simulink model "PRO_TestHarness"  (Simulink 8.6)
settings: Solver=ode45  StartTime=0.0  StopTime=10.0  RelTol=1e-3
PreLoadFcn:
  | addpath('./Workspace/')
  | load('./Workspace/EnvVar.mat')
  | if exist('tl_preloadfcn','file'), tl_preloadfcn(gcs,402); end
PostLoadFcn:
  | if exist('tl_postloadfcn','file'), tl_postloadfcn(gcs,402); end
InitFcn:
  | if exist('tlds_init','file'), tlds_init(gcs); end
StartFcn:
  | if exist('tlds_start','file'), tlds_start(gcs); end
StopFcn:
  | if exist('tlds_stop','file'), tlds_stop(gcs); end
undefined symbols (not defined in the file or in its folder): ddv, sigbuilder_block, Ts
libraries: tllib x19, simulink x2
(part 1 of 5)
PreSaveFcn:
  | if exist('tl_presavefcn','file'), tl_presavefcn(gcs); end
CloseFcn:
  | if exist('tl_closefcn','file'), tl_closefcn(gcs); end
settings Model: TL_MAIN_DATA={'codeopt',{'cleancode',1},'logopt',{'globalloggingmode',4},'date',736811.3266045833,'codegenerationmode',2}  TLRevision=402  DS_PROJECTFILE=PRO_TestHarness.dd  Creator=sabine.flechelle  LastModifiedBy=audrey.vache
settings DataIOCC: SignalLoggingSaveFormat=Dataset
settings OptimizationCC: BlockReduction=off  OptimizeBlockIOStorage=off  BufferReuse=off  GlobalBufferReuse=off  ExpressionFolding=off  ExpressionDepthLimit=128  LocalBlockOutputs=off
settings DebuggingCC: FcnCallInpInsideContextMsg=UseLocalSettings  BusObjectLabelMismatch=error  StateNameClashWarn=none  StrictBusMsg=ErrorOnBusTreatedAsVector  NonBusSignalsTreatedAsBus=error

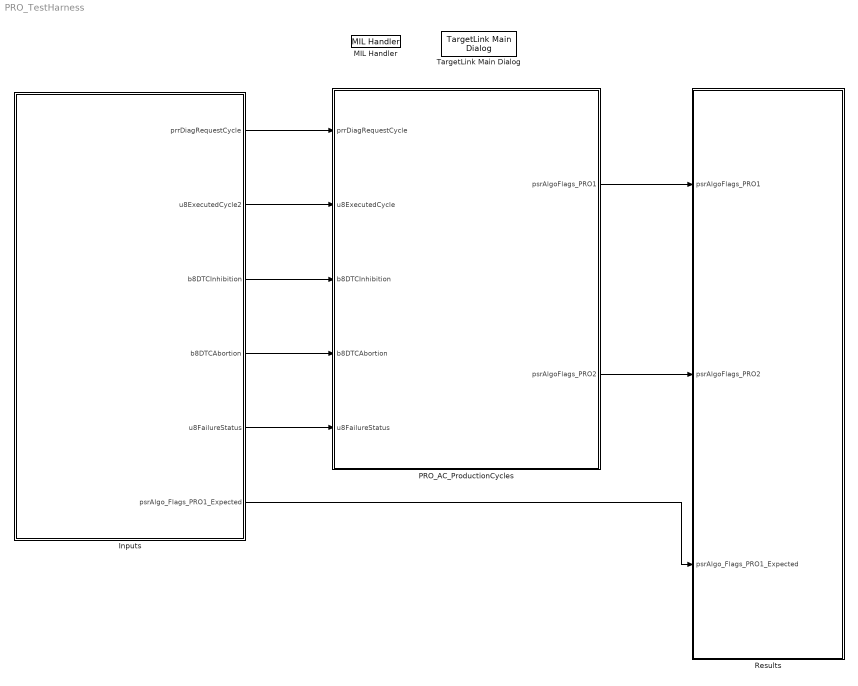
== system PRO_TestHarness ==
  Inputs : Subsystem
  MIL Handler : tllib/MIL Handler  data={'date',730486}
  PRO_AC_ProductionCycles : Subsystem  Tag=TargetLink Simulation Frame  mask(TL_SimFrame){}
      settings: CopyFcn=if exist('tl_copyfcn','file'), tl_copyfcn(gcbh); end  NameChangeFcn=if exist('tl_framenamechangefcn','file'), tl_framenamechangefcn(gcbh); end
      settings: OpenFcn=|
      | if exist('open_tlsubsystem','file')
      |    open_tlsubsystem(gcbh);
      | else
      |    tlsubsystem = ...
      |       find_system(gcb, ...
      |       'LookUnderMasks','on', ...
      |       'FollowLinks','on', ...
      |       'Tag','MIL Subsystem');
      |    open_system(tlsubsystem);
      | end
      mask Display: disp('TargetLink\nSoftware-\nin-the-loop\nmode')
  Results : Subsystem
  TargetLink Main Dialog : tllib/TargetLink Main Dialog  data=[]
  wires:
  Inputs/3(b8DTCInhibition) -> PRO_AC_ProductionCycles/3(b8DTCInhibition)
  Inputs/4(b8DTCAbortion) -> PRO_AC_ProductionCycles/4(b8DTCAbortion)
  Inputs/2(u8ExecutedCycle2) -> PRO_AC_ProductionCycles/2(u8ExecutedCycle)
  PRO_AC_ProductionCycles/1(psrAlgoFlags_PRO1) -> Results/1(psrAlgoFlags_PRO1)
  Inputs/6(psrAlgo_Flags_PRO1_Expected) -> Results/3(psrAlgo_Flags_PRO1_Expected)
  Inputs/1(prrDiagRequestCycle) -> PRO_AC_ProductionCycles/1(prrDiagRequestCycle)
  PRO_AC_ProductionCycles/2(psrAlgoFlags_PRO2) -> Results/2(psrAlgoFlags_PRO2)
  Inputs/5(u8FailureStatus) -> PRO_AC_ProductionCycles/5(u8FailureStatus)

== system PRO_TestHarness/Inputs ==
  Bus Creator1 : BusCreator  Inputs=2
  Bus Creator3 : BusCreator  Inputs=1
  BusCreator : BusCreator  Inputs=5
  Constant1 : Constant  Value=ddv('BFD/KU8_ZERO')  OutDataTypeStr=uint8  mask(TL_Constant){data={'output',{'variable','BFD/KU8_ZERO'},'date',736231.40062822914}}
      settings: DeleteFcn=if exist('delete_tlblock','file')==2,delete_tlblock(gcbh);end  NameChangeFcn=if exist('rename_tlblock','file')==2,rename_tlblock(gcbh);end  OpenFcn=if exist('tl_open_blockdlg','file')==2,tl_open_blockdlg(gcbh);else,open_system(gcbh,'parameter');end
      mask Help: eval(['if exist(''tl_online_help'',''file'') == 2, tl_online_help(''Topic'',''TL_Constant''),else, web([''jar:file:///'',matlabroot,''/help/toolbox/simulink/help.jar!/slref/' lower(get_param(gcbh,'Blocktype')) '.html''], ''-helpbrowser''),end'])
      mask Display: plot([-0.05, 1.05, NaN, -0.05, 1.05],[.01, .01, NaN, .99, .99])
  Manage_Sampling : Subsystem  TreatAsAtomicUnit=on
  Signal Builder : Subsystem  Tag=STV Subsys  LoadFcn=sigbuilder_block('load');  StartFcn=sigbuilder_block('start');  StopFcn=sigbuilder_block('stop');  ClipboardFcn=sigbuilder_block('clipboard');  mask(Sigbuilder block){}
      mask init:
      | if ~strcmp(get_param(bdroot(gcb),'SimulationStatus'),'stopped') tuvar = sigbuilder_block('maskInit'); end
      settings: CopyFcn=sigbuilder_block('copy');  DeleteFcn=sigbuilder_block('delete');  ModelCloseFcn=sigbuilder_block('modelClose');  PreSaveFcn=sigbuilder_block('preSave');  PauseFcn=sigbuilder_block('pause')  ContinueFcn=sigbuilder_block('continue')  NameChangeFcn=sigbuilder_block('namechange');  OpenFcn=sigbuilder_block('open',[132.75 123 813.75 406.5 ]);  CloseFcn=sigbuilder_block('close');
      mask Display: plot(0,0,100,100,[10,10,40,40,10],[80,20,20,80,80],[40,10],[50,50], [40,27,10],[65,72,56],[40,25,25,10],[28,28,43,43]);
  Terminator : Terminator
  prrDiagRequestCycle : Outport
  u8ExecutedCycle2 : Outport  Port=2  OutDataTypeStr=uint8  PortDimensions=1
  b8DTCInhibition : Outport  Port=3  PortDimensions=1
  b8DTCAbortion : Outport  Port=4  PortDimensions=1
  u8FailureStatus : Outport  Port=5
  psrAlgo_Flags_PRO1_Expected : Outport  Port=6
  wires:
  Manage_Sampling/4(b8DTCInhibition) -> b8DTCInhibition/1
  Manage_Sampling/3(u8ExecutedCycle2) -> u8ExecutedCycle2/1
  Manage_Sampling/5(b8DTCAbortion) -> b8DTCAbortion/1
  Bus Creator3/1 -> prrDiagRequestCycle/1
  Manage_Sampling/1(u8RequestedCycle1) -> Bus Creator3/1  "u8RequestedCycle"
  Manage_Sampling/2(u8RequestedCycleComplement1) -> Terminator/1  "u8RequestedCycleComplement"
  BusCreator/1 -> psrAlgo_Flags_PRO1_Expected/1
  Manage_Sampling/7(b8TriggeringOrder_Expected2) -> BusCreator/1
  Manage_Sampling/8(b8AbortionOrder_Expected2) -> BusCreator/2
  Manage_Sampling/9(b8PreActivationFlag_Expected1) -> BusCreator/3
  Manage_Sampling/10(b8PreConditionsFlag_Expected) -> BusCreator/4
  Manage_Sampling/11(u8TriggeringSource_Expected5) -> BusCreator/5
  Signal Builder/11(u8TriggeringSource_PRO1_Expected) -> Manage_Sampling/11(u8TriggeringSource_Expected4)
  Signal Builder/10(b8PreConditionsFlag_PRO1_Expected) -> Manage_Sampling/10(b8PreConditionsFlag_Expected2)
  Signal Builder/5(bAbortionMode) -> Manage_Sampling/5(b8DTCAbortion1)
  Signal Builder/3(u8ExecutedCycle) -> Manage_Sampling/3(u8ExecutedCycle)
  Signal Builder/4(btInhibitionMode) -> Manage_Sampling/4(b8DTCInhibition1)
  Signal Builder/8(b8AbortionFlag_PRO1_Expected) -> Manage_Sampling/8(b8AbortionOrder_Expected)
  Signal Builder/7(b8TriggerFlag_PRO1_Expected) -> Manage_Sampling/7(b8TriggeringOrder_Expected)
  Signal Builder/2(u8RequestedCycleComplement) -> Manage_Sampling/2(u8RequestedCycleComplement)
  Signal Builder/9(b8PreActivationFlag_PRO1_Expected) -> Manage_Sampling/9(b8PreActivationFlag_Expected)
  Signal Builder/1(u8RequestedCycle) -> Manage_Sampling/1(u8RequestedCycle)
  Bus Creator1/1 -> u8FailureStatus/1
  Constant1/1 -> Bus Creator1/1  "u8Status_UVDuringTensioning"
  Manage_Sampling/6(b8OverVoltageStatus1) -> Bus Creator1/2  "u8Status_OverVoltage"
  Signal Builder/6(b8OverVoltageStatus) -> Manage_Sampling/6(b8OverVoltageStatus)

== system PRO_TestHarness/PRO_AC_ProductionCycles ==
  prrDiagRequestCycle : Inport
  u8ExecutedCycle : Inport  Port=2
  b8DTCInhibition : Inport  Port=3  OutDataTypeStr=uint8
  b8DTCAbortion : Inport  Port=4  OutDataTypeStr=uint8
  u8FailureStatus : Inport  Port=5
  S-function frame : Subsystem
  Subsystem : Subsystem  Tag=struct('sfcnName','PRO_AC_ProductionCycles_sf','subFunction','','srcSubsystem','')  Commented=on  mask(TL_Enable){}
      settings: OpenFcn=warndlg(get_param(gcb,'MaskHelp'),'Serious Warning');
      mask Help: This subsystem keeps the TargetLink subsystem (subsystem with TargetLink blocks for production code generation), and is needed for the TargetLink simulation frame to work properly. DO NOT DELETE OR MODIFY IT!
  Timer : simulink/Ports & Subsystems/Function-Call Generator  sample_time=0.01  numberOfIterations=1
  psrAlgoFlags_PRO1 : Outport
  psrAlgoFlags_PRO2 : Outport  Port=2
  wires:
  Timer/1 -> S-function frame/Trigger
  prrDiagRequestCycle/1 -> S-function frame/1(In1)
  u8ExecutedCycle/1 -> S-function frame/2(In2)
  b8DTCInhibition/1 -> S-function frame/3(In3)
  b8DTCAbortion/1 -> S-function frame/4(In4)
  u8FailureStatus/1 -> S-function frame/5(In5)
  S-function frame/1(Out1) -> psrAlgoFlags_PRO1/1
  S-function frame/2(Out2) -> psrAlgoFlags_PRO2/1

== system PRO_TestHarness/Results ==
  psrAlgoFlags_PRO1 : Inport
  psrAlgoFlags_PRO2 : Inport  Port=2
  psrAlgo_Flags_PRO1_Expected : Inport  Port=3
  BusSelector1 : BusSelector  OutputSignals=b8TriggerFlag_PR01,b8InterruptFlag_PRO1,b8PreActivationFlag_PRO1,b8PreConditionsFlag_PRO1,u8TriggeringSource_PRO1
  BusSelector3 : BusSelector  OutputSignals=b8TriggerFlag_PRO2,b8InterruptFlag_PRO2,b8ActivationFlag_PRO2,b8PreConditionsFlag_PRO2,u8TriggeringSource_PRO2
  Data Type Conversion{,1,4,8..12,19..20} (10 alike) : DataTypeConversion  OutDataTypeStr=double  RndMeth=Nearest
  Mux : Mux  Inputs=10
  Scope : Scope  NumInputPorts=5
  To Workspace : ToWorkspace  VariableName=Simout  SaveFormat=Structure  SampleTime=-1
  wires:
  psrAlgoFlags_PRO1/1 -> BusSelector1/1
  BusSelector1/1 -> Scope/1, Data Type Conversion/1  "<b8TriggerFlag_PR01>"
  BusSelector1/2 -> Scope/2, Data Type Conversion1/1  "<b8InterruptFlag_PRO1>"
  Data Type Conversion/1 -> Mux/1
  Data Type Conversion1/1 -> Mux/2
  Data Type Conversion4/1 -> Mux/3
  Mux/1 -> To Workspace/1
  Data Type Conversion19/1 -> Mux/4
  Data Type Conversion20/1 -> Mux/5
  BusSelector1/3 -> Scope/3, Data Type Conversion4/1  "<b8PreActivationFlag_PRO1>"
  BusSelector1/4 -> Scope/4, Data Type Conversion19/1  "<b8PreConditionsFlag_PRO1>"
  BusSelector1/5 -> Scope/5, Data Type Conversion20/1  "<u8TriggeringSource_PRO1>"
  BusSelector3/1 -> Data Type Conversion8/1  "<b8TriggerFlag_PRO2>"
  BusSelector3/2 -> Data Type Conversion9/1  "<b8InterruptFlag_PRO2>"
  BusSelector3/3 -> Data Type Conversion12/1  "<b8ActivationFlag_PRO2>"
  BusSelector3/4 -> Data Type Conversion10/1  "<b8PreConditionsFlag_PRO2>"
  BusSelector3/5 -> Data Type Conversion11/1  "<u8TriggeringSource_PRO2>"
  psrAlgoFlags_PRO2/1 -> BusSelector3/1
  Data Type Conversion9/1 -> Mux/7
  Data Type Conversion8/1 -> Mux/6
  Data Type Conversion10/1 -> Mux/9
  Data Type Conversion11/1 -> Mux/10
  Data Type Conversion12/1 -> Mux/8

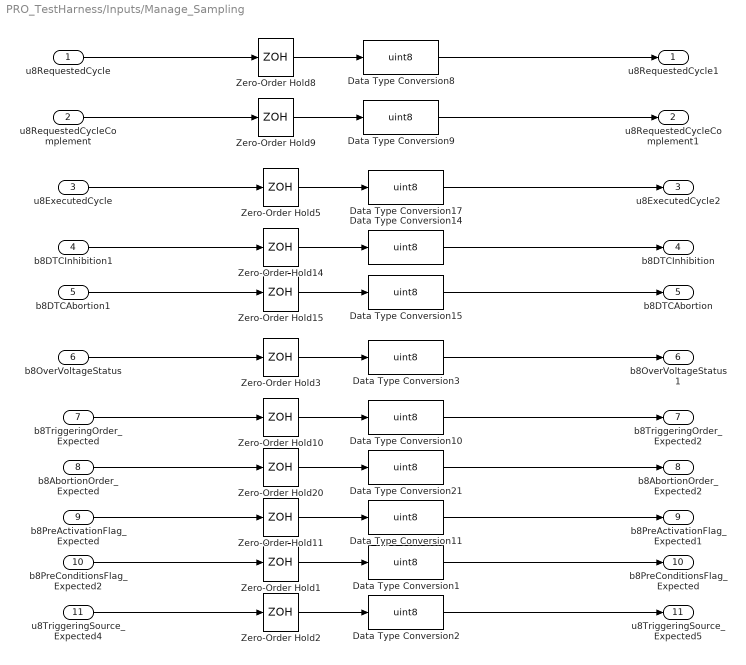
== system PRO_TestHarness/Inputs/Manage_Sampling ==
  u8RequestedCycle : Inport
      settings: NameChangeFcn=if exist('tl_check_ports','file'), tl_check_ports(gcbh); end
      settings: CopyFcn=|
      | if exist('tl_reset_reviewflag','file')==2
      |     tl_reset_reviewflag(gcbh);
      | end
      | if exist('tl_check_ports','file')
      |     tl_check_ports(gcbh);
      | end
  u8RequestedCycleComplement : Inport  Port=2
      settings: NameChangeFcn=if exist('tl_check_ports','file'), tl_check_ports(gcbh); end
      settings: CopyFcn=|
      | if exist('tl_reset_reviewflag','file')==2
      |     tl_reset_reviewflag(gcbh);
      | end
      | if exist('tl_check_ports','file')
      |     tl_check_ports(gcbh);
      | end
  u8ExecutedCycle : Inport  Port=3
      settings: NameChangeFcn=if exist('tl_check_ports','file'), tl_check_ports(gcbh); end
      settings: CopyFcn=|
      | if exist('tl_reset_reviewflag','file')==2
      |     tl_reset_reviewflag(gcbh);
      | end
      | if exist('tl_check_ports','file')
      |     tl_check_ports(gcbh);
      | end
  b8DTCInhibition1 : Inport  Port=4
      settings: NameChangeFcn=if exist('tl_check_ports','file'), tl_check_ports(gcbh); end
      settings: CopyFcn=|
      | if exist('tl_reset_reviewflag','file')==2
      |     tl_reset_reviewflag(gcbh);
      | end
      | if exist('tl_check_ports','file')
      |     tl_check_ports(gcbh);
      | end
  b8DTCAbortion1 : Inport  Port=5
      settings: NameChangeFcn=if exist('tl_check_ports','file'), tl_check_ports(gcbh); end
      settings: CopyFcn=|
      | if exist('tl_reset_reviewflag','file')==2
      |     tl_reset_reviewflag(gcbh);
      | end
      | if exist('tl_check_ports','file')
      |     tl_check_ports(gcbh);
      | end
  b8OverVoltageStatus : Inport  Port=6
      settings: NameChangeFcn=if exist('tl_check_ports','file'), tl_check_ports(gcbh); end
      settings: CopyFcn=|
      | if exist('tl_reset_reviewflag','file')==2
      |     tl_reset_reviewflag(gcbh);
      | end
      | if exist('tl_check_ports','file')
      |     tl_check_ports(gcbh);
      | end
  b8TriggeringOrder_Expected : Inport  Port=7
  b8AbortionOrder_Expected : Inport  Port=8
  b8PreActivationFlag_Expected : Inport  Port=9
  b8PreConditionsFlag_Expected2 : Inport  Port=10
  u8TriggeringSource_Expected4 : Inport  Port=11
  Data Type Conversion{1..3,8..11,14..15,17,21} (11 alike) : DataTypeConversion  OutDataTypeStr=uint8
  Zero-Order Hold{1..3,5,8..11,14..15,20} (11 alike) : ZeroOrderHold  SampleTime=Ts
  u8RequestedCycle1 : Outport  PortDimensions=1
  u8RequestedCycleComplement1 : Outport  Port=2  PortDimensions=1
  u8ExecutedCycle2 : Outport  Port=3  PortDimensions=1
  b8DTCInhibition : Outport  Port=4  PortDimensions=1
  b8DTCAbortion : Outport  Port=5  PortDimensions=1
  b8OverVoltageStatus1 : Outport  Port=6  PortDimensions=1
  b8TriggeringOrder_Expected2 : Outport  Port=7
  b8AbortionOrder_Expected2 : Outport  Port=8
  b8PreActivationFlag_Expected1 : Outport  Port=9
  b8PreConditionsFlag_Expected : Outport  Port=10
  u8TriggeringSource_Expected5 : Outport  Port=11
  wires:
  Data Type Conversion15/1 -> b8DTCAbortion/1
  Data Type Conversion14/1 -> b8DTCInhibition/1
  b8DTCAbortion1/1 -> Zero-Order Hold15/1
  Zero-Order Hold15/1 -> Data Type Conversion15/1
  b8DTCInhibition1/1 -> Zero-Order Hold14/1
  Zero-Order Hold14/1 -> Data Type Conversion14/1
  Data Type Conversion17/1 -> u8ExecutedCycle2/1
  u8ExecutedCycle/1 -> Zero-Order Hold5/1
  Zero-Order Hold5/1 -> Data Type Conversion17/1
  Zero-Order Hold10/1 -> Data Type Conversion10/1
  Zero-Order Hold11/1 -> Data Type Conversion11/1
  b8TriggeringOrder_Expected/1 -> Zero-Order Hold10/1
  Data Type Conversion10/1 -> b8TriggeringOrder_Expected2/1
  Zero-Order Hold20/1 -> Data Type Conversion21/1
  Data Type Conversion11/1 -> b8PreActivationFlag_Expected1/1
  Data Type Conversion21/1 -> b8AbortionOrder_Expected2/1
  b8AbortionOrder_Expected/1 -> Zero-Order Hold20/1
  b8PreActivationFlag_Expected/1 -> Zero-Order Hold11/1
  Data Type Conversion8/1 -> u8RequestedCycle1/1
  u8RequestedCycle/1 -> Zero-Order Hold8/1
  Zero-Order Hold8/1 -> Data Type Conversion8/1
  Data Type Conversion9/1 -> u8RequestedCycleComplement1/1
  u8RequestedCycleComplement/1 -> Zero-Order Hold9/1
  Zero-Order Hold9/1 -> Data Type Conversion9/1
  Zero-Order Hold1/1 -> Data Type Conversion1/1
  Data Type Conversion1/1 -> b8PreConditionsFlag_Expected/1
  b8PreConditionsFlag_Expected2/1 -> Zero-Order Hold1/1
  Zero-Order Hold2/1 -> Data Type Conversion2/1
  Data Type Conversion2/1 -> u8TriggeringSource_Expected5/1
  u8TriggeringSource_Expected4/1 -> Zero-Order Hold2/1
  Data Type Conversion3/1 -> b8OverVoltageStatus1/1
  b8OverVoltageStatus/1 -> Zero-Order Hold3/1
  Zero-Order Hold3/1 -> Data Type Conversion3/1

== system PRO_TestHarness/Inputs/Signal Builder ==
  Demux : Demux  Tag=STV Demux  Outputs=11
  FromWs : FromWorkspace  Tag=STV FromWs  VariableName=tuvar  SampleTime=0.01  Interpolate=off  OutputAfterFinalValue=Holding final value  SigBuilderData=DataTag0  VnvData=DataTag1
      SigBuilderData=|
      | dataSet(1).timeRange = [0 10]
      | dataSet(1).name = 'Template_Tests'
      | dataSet(2).timeRange = [0 10]
      | dataSet(2).name = 'MBD_PRO_01_Nominal'
      | dataSet(3).timeRange = [0 10]
      | dataSet(3).name = 'MBD_PRO_01_Nominal1'
      | dataSet(4).timeRange = [0 10]
      | dataSet(4).name = 'MBD_PRO_01_Nominal2'
      | sbobj.Name = 'Signal Builder'
      | sbobj.Groups(1).Name = 'Template_Tests'
      | sbobj.Groups(1).Signals(1).Name = 'u8RequestedCycle'
      | sbobj.Groups(1).Signals(1).XData = [0 10]
      | sbobj.Groups(1).Signals(1).YData = [0 0]
      | sbobj.Groups(1).Signals(2).Name = 'u8RequestedCycleComplement'
      | sbobj.Groups(1).Signals(2).XData = [0 10]
      | sbobj.Groups(1).Signals(2).YData = [0 0]
      | sbobj.Groups(1).Signals(3).Name = 'u8ExecutedCycle'
      | sbobj.Groups(1).Signals(3).XData = [0 10]
      | sbobj.Groups(1).Signals(3).YData = [0 0]
      | sbobj.Groups(1).Signals(4).Name = 'btInhibitionMode'
      | sbobj.Groups(1).Signals(4).XData = [0 10]
      | sbobj.Groups(1).Signals(4).YData = [0 0]
      | sbobj.Groups(1).Signals(5).Name = 'bAbortionMode'
      | sbobj.Groups(1).Signals(5).XData = [0 10]
      | sbobj.Groups(1).Signals(5).YData = [0 0]
      | sbobj.Groups(1).Signals(6).Name = 'b8OverVoltageStatus'
      | sbobj.Groups(1).Signals(6).XData = [0 10]
      | sbobj.Groups(1).Signals(6).YData = [0 0]
      | sbobj.Groups(1).Signals(7).Name = 'b8TriggerFlag_PRO1_Expected'
      | sbobj.Groups(1).Signals(7).XData = [0 10]
      | sbobj.Groups(1).Signals(7).YData = [0 0]
      | sbobj.Groups(1).Signals(8).Name = 'b8AbortionFlag_PRO1_Expected'
      | sbobj.Groups(1).Signals(8).XData = [0 10]
      | sbobj.Groups(1).Signals(8).YData = [0 0]
      | sbobj.Groups(1).Signals(9).Name = 'b8PreActivationFlag_PRO1_Expected'
      | sbobj.Groups(1).Signals(9).XData = [0 10]
      | sbobj.Groups(1).Signals(9).YData = [0 0]
      | sbobj.Groups(1).Signals(10).Name = 'b8PreConditionsFlag_PRO1_Expected'
      | sbobj.Groups(1).Signals(10).XData = [0 10]
      | sbobj.Groups(1).Signals(10).YData = [0 0]
      | sbobj.Groups(1).Signals(11).Name = 'u8TriggeringSource_PRO1_Expected'
      | sbobj.Groups(1).Signals(11).XData = [0 10]
      | sbobj.Groups(1).Signals(11).YData = [0 0]
      | sbobj.Groups(2).Name = 'MBD_PRO_01_Nominal'
      | sbobj.Groups(2).Signals(1).Name = 'u8RequestedCycle'
      | sbobj.Groups(2).Signals(1).XData = [0 0.009 0.009 0.019 0.019 0.029 0.029 0.039 0.039 0.049 0.049 0.059 ... (2000 elements, 1x2000)]
      | sbobj.Groups(2).Signals(1).YData = [255 255 255 255 255 255 255 255 255 255 255 255 ... (2000 elements, 1x2000)]
      | sbobj.Groups(2).Signals(2).Name = 'u8RequestedCycleComplement'
      | sbobj.Groups(2).Signals(2).XData = [0 0.009 0.009 0.019 0.019 0.029 0.029 0.039 0.039 0.049 0.049 0.059 ... (2000 elements, 1x2000)]
      | sbobj.Groups(2).Signals(2).YData = [0 0 0 0 0 0 0 0 0 0 0 0 ... (2000 elements, 1x2000)]
      | sbobj.Groups(2).Signals(3).Name = 'u8ExecutedCycle'
      | sbobj.Groups(2).Signals(3).XData = [0 0.009 0.009 0.019 0.019 0.029 0.029 0.039 0.039 0.049 0.049 0.059 ... (2000 elements, 1x2000)]
      | sbobj.Groups(2).Signals(3).YData = [255 255 255 255 255 255 255 255 255 255 255 255 ... (2000 elements, 1x2000)]
      | sbobj.Groups(2).Signals(4).Name = 'btInhibitionMode'
      | sbobj.Groups(2).Signals(4).XData = [0 0.009 0.009 0.019 0.019 0.029 0.029 0.039 0.039 0.049 0.049 0.059 ... (2000 elements, 1x2000)]
      | sbobj.Groups(2).Signals(4).YData = [85 85 85 85 85 85 85 85 85 85 85 85 ... (2000 elements, 1x2000)]
      | sbobj.Groups(2).Signals(5).Name = 'bAbortionMode'
      | sbobj.Groups(2).Signals(5).XData = [0 0.009 0.009 0.019 0.019 0.029 0.029 0.039 0.039 0.049 0.049 0.059 ... (2000 elements, 1x2000)]
      | sbobj.Groups(2).Signals(5).YData = [85 85 85 85 85 85 85 85 85 85 85 85 ... (2000 elements, 1x2000)]
      | sbobj.Groups(2).Signals(6).Name = 'b8OverVoltageStatus'
      | sbobj.Groups(2).Signals(6).XData = [0 0.009 0.009 0.019 0.019 0.029 0.029 0.039 0.039 0.049 0.049 0.059 ... (2000 elements, 1x2000)]
      | sbobj.Groups(2).Signals(6).YData = [0 0 0 0 0 0 0 0 0 0 0 0 ... (2000 elements, 1x2000)]
      | sbobj.Groups(2).Signals(7).Name = 'b8TriggerFlag_PRO1_Expected'
      | sbobj.Groups(2).Signals(7).XData = [0 0.009 0.009 0.019 0.019 0.029 0.029 0.039 0.039 0.049 0.049 0.059 ... (2000 elements, 1x2000)]
      | sbobj.Groups(2).Signals(7).YData = [85 85 85 85 85 85 85 85 85 85 85 85 ... (2000 elements, 1x2000)]
      | sbobj.Groups(2).Signals(8).Name = 'b8AbortionFlag_PRO1_Expected'
      | sbobj.Groups(2).Signals(8).XData = [0 0.009 0.009 0.019 0.019 0.029 0.029 0.039 0.039 0.049 0.049 0.059 ... (2000 elements, 1x2000)]
      | sbobj.Groups(2).Signals(8).YData = [85 85 85 85 85 85 85 85 85 85 85 85 ... (2000 elements, 1x2000)]
      | sbobj.Groups(2).Signals(9).Name = 'b8PreActivationFlag_PRO1_Expected'
      | sbobj.Groups(2).Signals(9).XData = [0 0.009 0.009 0.019 0.019 0.029 0.029 0.039 0.039 0.049 0.049 0.059 ... (2000 elements, 1x2000)]
      | sbobj.Groups(2).Signals(9).YData = [85 85 85 85 85 85 85 85 85 85 85 85 ... (2000 elements, 1x2000)]
      | sbobj.Groups(2).Signals(10).Name = 'b8PreConditionsFlag_PRO1_Expected'
      | sbobj.Groups(2).Signals(10).XData = [0 0.009 0.009 0.019 0.019 0.029 0.029 0.039 0.039 0.049 0.049 0.059 ... (2000 elements, 1x2000)]
      | sbobj.Groups(2).Signals(10).YData = [170 170 170 170 170 170 170 170 170 170 170 170 ... (2000 elements, 1x2000)]
      | sbobj.Groups(2).Signals(11).Name = 'u8TriggeringSource_PRO1_Expected'
      | sbobj.Groups(2).Signals(11).XData = [0 0.009 0.009 0.019 0.019 0.029 0.029 0.039 0.039 0.049 0.049 0.059 ... (2000 elements, 1x2000)]
      | sbobj.Groups(2).Signals(11).YData = [0 0 0 0 0 0 0 0 0 0 0 0 ... (2000 elements, 1x2000)]
      | sbobj.Groups(3).Name = 'MBD_PRO_01_Nominal1'
      | sbobj.Groups(3).Signals(1).Name = 'u8RequestedCycle'
      | sbobj.Groups(3).Signals(1).XData = [0 0.009 0.009 0.019 0.019 0.029 0.029 0.039 0.039 0.049 0.049 0.059 ... (2000 elements, 1x2000)]
      | sbobj.Groups(3).Signals(1).YData = [255 255 255 255 255 255 255 255 255 255 255 255 ... (2000 elements, 1x2000)]
      | sbobj.Groups(3).Signals(2).Name = 'u8RequestedCycleComplement'
      | sbobj.Groups(3).Signals(2).XData = [0 0.009 0.009 0.019 0.019 0.029 0.029 0.039 0.039 0.049 0.049 0.059 ... (2000 elements, 1x2000)]
      | sbobj.Groups(3).Signals(2).YData = [0 0 0 0 0 0 0 0 0 0 0 0 ... (2000 elements, 1x2000)]
      | sbobj.Groups(3).Signals(3).Name = 'u8ExecutedCycle'
      | sbobj.Groups(3).Signals(3).XData = [0 0.009 0.009 0.019 0.019 0.029 0.029 0.039 0.039 0.049 0.049 0.059 ... (2000 elements, 1x2000)]
      | sbobj.Groups(3).Signals(3).YData = [255 255 255 255 255 255 255 255 255 255 255 255 ... (2000 elements, 1x2000)]
      | sbobj.Groups(3).Signals(4).Name = 'btInhibitionMode'
      | sbobj.Groups(3).Signals(4).XData = [0 0.009 0.009 0.019 0.019 0.029 0.029 0.039 0.039 0.049 0.049 0.059 ... (2000 elements, 1x2000)]
      | sbobj.Groups(3).Signals(4).YData = [85 85 85 85 85 85 85 85 85 85 85 85 ... (2000 elements, 1x2000)]
      | sbobj.Groups(3).Signals(5).Name = 'bAbortionMode'
      | sbobj.Groups(3).Signals(5).XData = [0 0.009 0.009 0.019 0.019 0.029 0.029 0.039 0.039 0.049 0.049 0.059 ... (2000 elements, 1x2000)]
      | sbobj.Groups(3).Signals(5).YData = [85 85 85 85 85 85 85 85 85 85 85 85 ... (2000 elements, 1x2000)]
      | sbobj.Groups(3).Signals(6).Name = 'b8OverVoltageStatus'
      | sbobj.Groups(3).Signals(6).XData = [0 0.009 0.009 0.019 0.019 0.029 0.029 0.039 0.039 0.049 0.049 0.059 ... (2000 elements, 1x2000)]
      | sbobj.Groups(3).Signals(6).YData = [0 0 0 0 0 0 0 0 0 0 0 0 ... (2000 elements, 1x2000)]
      | sbobj.Groups(3).Signals(7).Name = 'b8TriggerFlag_PRO1_Expected'
      | sbobj.Groups(3).Signals(7).XData = [0 0.009 0.009 0.019 0.019 0.029 0.029 0.039 0.039 0.049 0.049 0.059 ... (2000 elements, 1x2000)]
      | sbobj.Groups(3).Signals(7).YData = [85 85 85 85 85 85 85 85 85 85 85 85 ... (2000 elements, 1x2000)]
      | sbobj.Groups(3).Signals(8).Name = 'b8AbortionFlag_PRO1_Expected'
      | sbobj.Groups(3).Signals(8).XData = [0 0.009 0.009 0.019 0.019 0.029 0.029 0.039 0.039 0.049 0.049 0.059 ... (2000 elements, 1x2000)]
      | sbobj.Groups(3).Signals(8).YData = [85 85 85 85 85 85 85 85 85 85 85 85 ... (2000 elements, 1x2000)]
      | sbobj.Groups(3).Signals(9).Name = 'b8PreActivationFlag_PRO1_Expected'
      | sbobj.Groups(3).Signals(9).XData = [0 0.009 0.009 0.019 0.019 0.029 0.029 0.039 0.039 0.049 0.049 0.059 ... (2000 elements, 1x2000)]
      | sbobj.Groups(3).Signals(9).YData = [85 85 85 85 85 85 85 85 85 85 85 85 ... (2000 elements, 1x2000)]
      | sbobj.Groups(3).Signals(10).Name = 'b8PreConditionsFlag_PRO1_Expected'
      | sbobj.Groups(3).Signals(10).XData = [0 0.009 0.009 0.019 0.019 0.029 0.029 0.039 0.039 0.049 0.049 0.059 ... (2000 elements, 1x2000)]
      | sbobj.Groups(3).Signals(10).YData = [170 170 170 170 170 170 170 170 170 170 170 170 ... (2000 elements, 1x2000)]
      | sbobj.Groups(3).Signals(11).Name = 'u8TriggeringSource_PRO1_Expected'
      | sbobj.Groups(3).Signals(11).XData = [0 0.009 0.009 0.019 0.019 0.029 0.029 0.039 0.039 0.049 0.049 0.059 ... (2000 elements, 1x2000)]
      | sbobj.Groups(3).Signals(11).YData = [0 0 0 0 0 0 0 0 0 0 0 0 ... (2000 elements, 1x2000)]
      | sbobj.Groups(4).Name = 'MBD_PRO_01_Nominal2'
      | sbobj.Groups(4).Signals(1).Name = 'u8RequestedCycle'
      | sbobj.Groups(4).Signals(1).XData = [0 0.009 0.009 0.019 0.019 0.029 0.029 0.039 0.039 0.049 0.049 0.059 ... (2000 elements, 1x2000)]
      | sbobj.Groups(4).Signals(1).YData = [255 255 255 255 255 255 255 255 255 255 255 255 ... (2000 elements, 1x2000)]
      | sbobj.Groups(4).Signals(2).Name = 'u8RequestedCycleComplement'
      | sbobj.Groups(4).Signals(2).XData = [0 0.009 0.009 0.019 0.019 0.029 0.029 0.039 0.039 0.049 0.049 0.059 ... (2000 elements, 1x2000)]
      | sbobj.Groups(4).Signals(2).YData = [0 0 0 0 0 0 0 0 0 0 0 0 ... (2000 elements, 1x2000)]
      | sbobj.Groups(4).Signals(3).Name = 'u8ExecutedCycle'
      | sbobj.Groups(4).Signals(3).XData = [0 0.009 0.009 0.019 0.019 0.029 0.029 0.039 0.039 0.049 0.049 0.059 ... (2000 elements, 1x2000)]
      | sbobj.Groups(4).Signals(3).YData = [255 255 255 255 255 255 255 255 255 255 255 255 ... (2000 elements, 1x2000)]
      | sbobj.Groups(4).Signals(4).Name = 'btInhibitionMode'
      | sbobj.Groups(4).Signals(4).XData = [0 0.009 0.009 0.019 0.019 0.029 0.029 0.039 0.039 0.049 0.049 0.059 ... (2000 elements, 1x2000)]
      | sbobj.Groups(4).Signals(4).YData = [85 85 85 85 85 85 85 85 85 85 85 85 ... (2000 elements, 1x2000)]
      | sbobj.Groups(4).Signals(5).Name = 'bAbortionMode'
      | sbobj.Groups(4).Signals(5).XData = [0 0.009 0.009 0.019 0.019 0.029 0.029 0.039 0.039 0.049 0.049 0.059 ... (2000 elements, 1x2000)]
      | sbobj.Groups(4).Signals(5).YData = [85 85 85 85 85 85 85 85 85 85 85 85 ... (2000 elements, 1x2000)]
      | sbobj.Groups(4).Signals(6).Name = 'b8OverVoltageStatus'
      | sbobj.Groups(4).Signals(6).XData = [0 0.009 0.009 0.019 0.019 0.029 0.029 0.039 0.039 0.049 0.049 0.059 ... (2000 elements, 1x2000)]
      | sbobj.Groups(4).Signals(6).YData = [0 0 0 0 0 0 0 0 0 0 0 0 ... (2000 elements, 1x2000)]
      | sbobj.Groups(4).Signals(7).Name = 'b8TriggerFlag_PRO1_Expected'
      | sbobj.Groups(4).Signals(7).XData = [0 0.009 0.009 0.019 0.019 0.029 0.029 0.039 0.039 0.049 0.049 0.059 ... (2000 elements, 1x2000)]
      | sbobj.Groups(4).Signals(7).YData = [85 85 85 85 85 85 85 85 85 85 85 85 ... (2000 elements, 1x2000)]
      | sbobj.Groups(4).Signals(8).Name = 'b8AbortionFlag_PRO1_Expected'
      | sbobj.Groups(4).Signals(8).XData = [0 0.009 0.009 0.019 0.019 0.029 0.029 0.039 0.039 0.049 0.049 0.059 ... (2000 elements, 1x2000)]
      | sbobj.Groups(4).Signals(8).YData = [85 85 85 85 85 85 85 85 85 85 85 85 ... (2000 elements, 1x2000)]
      | sbobj.Groups(4).Signals(9).Name = 'b8PreActivationFlag_PRO1_Expected'
      | sbobj.Groups(4).Signals(9).XData = [0 0.009 0.009 0.019 0.019 0.029 0.029 0.039 0.039 0.049 0.049 0.059 ... (2000 elements, 1x2000)]
      | sbobj.Groups(4).Signals(9).YData = [85 85 85 85 85 85 85 85 85 85 85 85 ... (2000 elements, 1x2000)]
      | sbobj.Groups(4).Signals(10).Name = 'b8PreConditionsFlag_PRO1_Expected'
      | sbobj.Groups(4).Signals(10).XData = [0 0.009 0.009 0.019 0.019 0.029 0.029 0.039 0.039 0.049 0.049 0.059 ... (2000 elements, 1x2000)]
      | sbobj.Groups(4).Signals(10).YData = [170 170 170 170 170 170 170 170 170 170 170 170 ... (2000 elements, 1x2000)]
      | sbobj.Groups(4).Signals(11).Name = 'u8TriggeringSource_PRO1_Expected'
      | sbobj.Groups(4).Signals(11).XData = [0 0.009 0.009 0.019 0.019 0.029 0.029 0.039 0.039 0.049 0.049 0.059 ... (2000 elements, 1x2000)]
      | sbobj.Groups(4).Signals(11).YData = [0 0 0 0 0 0 0 0 0 0 0 0 ... (2000 elements, 1x2000)]
  u8RequestedCycle : Outport  Tag=STV Outport
  u8RequestedCycleComplement : Outport  Tag=STV Outport  Port=2
  u8ExecutedCycle : Outport  Tag=STV Outport  Port=3
  btInhibitionMode : Outport  Tag=STV Outport  Port=4
  bAbortionMode : Outport  Tag=STV Outport  Port=5
  b8OverVoltageStatus : Outport  Tag=STV Outport  Port=6
  b8TriggerFlag_PRO1_Expected : Outport  Tag=STV Outport  Port=7
  b8AbortionFlag_PRO1_Expected : Outport  Tag=STV Outport  Port=8
  b8PreActivationFlag_PRO1_Expected : Outport  Tag=STV Outport  Port=9
  b8PreConditionsFlag_PRO1_Expected : Outport  Tag=STV Outport  Port=10
  u8TriggeringSource_PRO1_Expected : Outport  Tag=STV Outport  Port=11
  wires:
  FromWs/1 -> Demux/1
  Demux/1 -> u8RequestedCycle/1
  Demux/2 -> u8RequestedCycleComplement/1
  Demux/3 -> u8ExecutedCycle/1
  Demux/4 -> btInhibitionMode/1
  Demux/5 -> bAbortionMode/1
  Demux/6 -> b8OverVoltageStatus/1
  Demux/7 -> b8TriggerFlag_PRO1_Expected/1
  Demux/8 -> b8AbortionFlag_PRO1_Expected/1
  Demux/9 -> b8PreActivationFlag_PRO1_Expected/1
  Demux/10 -> b8PreConditionsFlag_PRO1_Expected/1
  Demux/11 -> u8TriggeringSource_PRO1_Expected/1

== system PRO_TestHarness/PRO_AC_ProductionCycles/S-function frame ==
  In1 : Inport
  In2 : Inport  Port=2
  In3 : Inport  Port=3  OutDataTypeStr=uint8
  In4 : Inport  Port=4  OutDataTypeStr=uint8
  In5 : Inport  Port=5
  TriggerPort : TriggerPort  TriggerType=function-call  ShowOutputPort=on
  Adaptor-In : Subsystem
  Adaptor-Out : Subsystem
  S-function : S-Function  Tag=FXP_HOST_SIM  InitFcn=clear pro_ac_productioncycles_sf  FunctionName=PRO_AC_ProductionCycles_sf  Parameters='PRO_TestHarness' , 'HostPC64' , 'GCC', 'HostPC'  SFunctionDeploymentMode=off  EnableBusSupport=off
  Out1 : Outport
  Out2 : Outport  Port=2
  wires:
  TriggerPort/1 -> S-function/1
  In1/1 -> Adaptor-In/1(In1)
  In2/1 -> Adaptor-In/2(In2)
  In3/1 -> Adaptor-In/3(In3)
  In4/1 -> Adaptor-In/4(In4)
  In5/1 -> Adaptor-In/5(In5)
  Adaptor-In/1(Out1) -> S-function/2
  Adaptor-In/2(Out2) -> S-function/3
  Adaptor-In/3(Out3) -> S-function/4
  Adaptor-In/4(Out4) -> S-function/5
  Adaptor-In/5(Out5) -> S-function/6
  Adaptor-In/6(Out6) -> S-function/7
  S-function/1 -> Adaptor-Out/1(In1)
  S-function/2 -> Adaptor-Out/2(In2)
  S-function/3 -> Adaptor-Out/3(In3)
  S-function/4 -> Adaptor-Out/4(In4)
  S-function/5 -> Adaptor-Out/5(In5)
  S-function/6 -> Adaptor-Out/6(In6)
  S-function/7 -> Adaptor-Out/7(In7)
  S-function/8 -> Adaptor-Out/8(In8)
  S-function/9 -> Adaptor-Out/9(In9)
  S-function/10 -> Adaptor-Out/10(In10)
  Adaptor-Out/1(Out1) -> Out1/1
  Adaptor-Out/2(Out2) -> Out2/1

== system PRO_TestHarness/PRO_AC_ProductionCycles/Subsystem ==
  prrDiagRequestCycle : Inport
  u8ExecutedCycle : Inport  Port=2
  b8DTCInhibition : Inport  Port=3  OutDataTypeStr=uint8
  b8DTCAbortion : Inport  Port=4  OutDataTypeStr=uint8
  u8FailureStatus : Inport  Port=5
  PRO_AC_ProductionCycles : Subsystem  Tag=disabled MIL Subsystem  Description=a  mask(MIL Subsystem){}
      settings: CopyFcn=if exist('tl_copyfcn','file'), tl_copyfcn(gcbh); end  NameChangeFcn=if exist('tl_namechangefcn','file'), tl_namechangefcn(gcbh); end  DestroyFcn=if exist('update_tl_main_dlg','file'), update_tl_main_dlg('TL_subs_display'); end
  psrAlgoFlags_PRO1 : Outport
  psrAlgoFlags_PRO2 : Outport  Port=2
  wires:
  PRO_AC_ProductionCycles/1(psrAlgoFlags_PRO1) -> psrAlgoFlags_PRO1/1
  PRO_AC_ProductionCycles/2(psrAlgoFlags_PRO2) -> psrAlgoFlags_PRO2/1
  prrDiagRequestCycle/1 -> PRO_AC_ProductionCycles/1(prrDiagRequestCycle)
  u8ExecutedCycle/1 -> PRO_AC_ProductionCycles/2(u8ExecutedCycle)
  b8DTCInhibition/1 -> PRO_AC_ProductionCycles/3(b8DTCInhibition)
  b8DTCAbortion/1 -> PRO_AC_ProductionCycles/4(b8DTCAbortion)
  u8FailureStatus/1 -> PRO_AC_ProductionCycles/5(u8FailureStatus)

== system PRO_TestHarness/PRO_AC_ProductionCycles/S-function frame/Adaptor-In ==
  In1 : Inport
  In2 : Inport  Port=2
  In3 : Inport  Port=3
  In4 : Inport  Port=4
  In5 : Inport  Port=5
  BusSelector1 : BusSelector  OutputSignals=u8RequestedCycle
  BusSelector5 : BusSelector  OutputSignals=u8Status_UVDuringTensioning,u8Status_OverVoltage
  Out1 : Outport
  Out2 : Outport  Port=2
  Out3 : Outport  Port=3
  Out4 : Outport  Port=4
  Out5 : Outport  Port=5
  Out6 : Outport  Port=6
  wires:
  BusSelector1/1 -> Out1/1  "<u8RequestedCycle>"
  In1/1 -> BusSelector1/1
  In2/1 -> Out2/1
  In3/1 -> Out3/1
  In4/1 -> Out4/1
  BusSelector5/1 -> Out5/1  "<u8Status_UVDuringTensioning>"
  BusSelector5/2 -> Out6/1  "<u8Status_OverVoltage>"
  In5/1 -> BusSelector5/1

== system PRO_TestHarness/PRO_AC_ProductionCycles/S-function frame/Adaptor-Out ==
  In1 : Inport
  In2 : Inport  Port=2
  In3 : Inport  Port=3
  In4 : Inport  Port=4
  In5 : Inport  Port=5
  In6 : Inport  Port=6
  In7 : Inport  Port=7
  In8 : Inport  Port=8
  In9 : Inport  Port=9
  In10 : Inport  Port=10
  BusCreator1_1 : BusCreator  Inputs=5
  BusCreator2_1 : BusCreator  Inputs=5
  Out1 : Outport
  Out2 : Outport  Port=2
  wires:
  In1/1 -> BusCreator1_1/1  "b8TriggerFlag_PR01"
  In2/1 -> BusCreator1_1/2  "b8InterruptFlag_PRO1"
  In3/1 -> BusCreator1_1/3  "b8PreActivationFlag_PRO1"
  In4/1 -> BusCreator1_1/4  "b8PreConditionsFlag_PRO1"
  In5/1 -> BusCreator1_1/5  "u8TriggeringSource_PRO1"
  BusCreator1_1/1 -> Out1/1
  In6/1 -> BusCreator2_1/1  "b8TriggerFlag_PRO2"
  In7/1 -> BusCreator2_1/2  "b8InterruptFlag_PRO2"
  In8/1 -> BusCreator2_1/3  "b8ActivationFlag_PRO2"
  In9/1 -> BusCreator2_1/4  "b8PreConditionsFlag_PRO2"
  In10/1 -> BusCreator2_1/5  "u8TriggeringSource_PRO2"
  BusCreator2_1/1 -> Out2/1

== system PRO_TestHarness/PRO_AC_ProductionCycles/Subsystem/PRO_AC_ProductionCycles ==
  prrDiagRequestCycle : Inport  mask(TL_BusInport){data={'signals',{{'',{'u8RequestedCycle'}}},'date',736042.68715741893}}
      settings: DeleteFcn=if exist('delete_tlblock','file')==2,delete_tlblock(gcbh);end  OpenFcn=if exist('tl_open_blockdlg','file')==2,tl_open_blockdlg(gcbh);else,open_system(gcbh,'parameter');end
      settings: CopyFcn=|
      | if exist('tl_reset_reviewflag','file')==2
      |     tl_reset_reviewflag(gcbh);
      | end
      | if exist('tl_check_ports','file')
      |     tl_check_ports(gcbh);
      | end
      settings: NameChangeFcn=|
      | if exist('rename_tlblock','file')==2,rename_tlblock(gcbh);end
      | if exist('tl_check_ports','file'), tl_check_ports(gcbh); end
      mask Help: eval(['if exist(''tl_online_help'',''file'') == 2, tl_online_help(''Topic'',''TL_Inport''),else, web([''jar:file:///'',matlabroot,''/help/toolbox/simulink/help.jar!/slref/' lower(get_param(gcbh,'Blocktype')) '.html''], ''-helpbrowser''),end'])
      mask Display: plot([0.2 0.35 NaN 0.65 0.8],[0 1 NaN 0 1]);
  u8ExecutedCycle : Inport  Port=2  mask(TL_Inport){data={'output',{'type','UInt8'},'date',735641.48482696759}}
      settings: DeleteFcn=if exist('delete_tlblock','file')==2,delete_tlblock(gcbh);end  OpenFcn=if exist('tl_open_blockdlg','file')==2,tl_open_blockdlg(gcbh);else,open_system(gcbh,'parameter');end
      settings: CopyFcn=|
      | if exist('tl_reset_reviewflag','file')==2
      |     tl_reset_reviewflag(gcbh);
      | end
      | if exist('tl_check_ports','file')
      |     tl_check_ports(gcbh);
      | end
      settings: NameChangeFcn=|
      | if exist('rename_tlblock','file')==2,rename_tlblock(gcbh);end
      | if exist('tl_check_ports','file'), tl_check_ports(gcbh); end
      mask Help: eval(['if exist(''tl_online_help'',''file'') == 2, tl_online_help(''Topic'',''TL_Inport''),else, web([''jar:file:///'',matlabroot,''/help/toolbox/simulink/help.jar!/slref/' lower(get_param(gcbh,'Blocktype')) '.html''], ''-helpbrowser''),end'])
      mask Display: plot([0.2 0.35 NaN 0.65 0.8],[0 1 NaN 0 1]);
  b8DTCInhibition : Inport  Port=3  OutDataTypeStr=uint8  mask(TL_Inport){data={'output',{'type','UInt8'},'date',735620.38775060186}}
      settings: DeleteFcn=if exist('delete_tlblock','file')==2,delete_tlblock(gcbh);end  OpenFcn=if exist('tl_open_blockdlg','file')==2,tl_open_blockdlg(gcbh);else,open_system(gcbh,'parameter');end
      settings: CopyFcn=|
      | if exist('tl_reset_reviewflag','file')==2
      |     tl_reset_reviewflag(gcbh);
      | end
      | if exist('tl_check_ports','file')
      |     tl_check_ports(gcbh);
      | end
      settings: NameChangeFcn=|
      | if exist('rename_tlblock','file')==2,rename_tlblock(gcbh);end
      | if exist('tl_check_ports','file'), tl_check_ports(gcbh); end
      mask Help: eval(['if exist(''tl_online_help'',''file'') == 2, tl_online_help(''Topic'',''TL_Inport''),else, web([''jar:file:///'',matlabroot,''/help/toolbox/simulink/help.jar!/slref/' lower(get_param(gcbh,'Blocktype')) '.html''], ''-helpbrowser''),end'])
      mask Display: plot([0.2 0.35 NaN 0.65 0.8],[0 1 NaN 0 1]);
  b8DTCAbortion : Inport  Port=4  OutDataTypeStr=uint8  mask(TL_Inport){data={'output',{'type','UInt8'},'date',735641.48518160882}}
      settings: DeleteFcn=if exist('delete_tlblock','file')==2,delete_tlblock(gcbh);end  OpenFcn=if exist('tl_open_blockdlg','file')==2,tl_open_blockdlg(gcbh);else,open_system(gcbh,'parameter');end
      settings: CopyFcn=|
      | if exist('tl_reset_reviewflag','file')==2
      |     tl_reset_reviewflag(gcbh);
      | end
      | if exist('tl_check_ports','file')
      |     tl_check_ports(gcbh);
      | end
      settings: NameChangeFcn=|
      | if exist('rename_tlblock','file')==2,rename_tlblock(gcbh);end
      | if exist('tl_check_ports','file'), tl_check_ports(gcbh); end
      mask Help: eval(['if exist(''tl_online_help'',''file'') == 2, tl_online_help(''Topic'',''TL_Inport''),else, web([''jar:file:///'',matlabroot,''/help/toolbox/simulink/help.jar!/slref/' lower(get_param(gcbh,'Blocktype')) '.html''], ''-helpbrowser''),end'])
      mask Display: plot([0.2 0.35 NaN 0.65 0.8],[0 1 NaN 0 1]);
  u8FailureStatus : Inport  Port=5  mask(TL_BusInport){data={'#autoscaling',2,'#message',2,'#output',2,'#logdata',2,'signals',{{'',{'u8Status_UVDuringTensioning';'u8Status_OverVoltage'}}},'date',735928.370256169}}
      settings: DeleteFcn=if exist('delete_tlblock','file')==2,delete_tlblock(gcbh);end  OpenFcn=if exist('tl_open_blockdlg','file')==2,tl_open_blockdlg(gcbh);else,open_system(gcbh,'parameter');end
      settings: CopyFcn=|
      | if exist('tl_reset_reviewflag','file')==2
      |     tl_reset_reviewflag(gcbh);
      | end
      | if exist('tl_check_ports','file')
      |     tl_check_ports(gcbh);
      | end
      settings: NameChangeFcn=|
      | if exist('rename_tlblock','file')==2,rename_tlblock(gcbh);end
      | if exist('tl_check_ports','file'), tl_check_ports(gcbh); end
      mask Help: eval(['if exist(''tl_online_help'',''file'') == 2, tl_online_help(''Topic'',''TL_Inport''),else, web([''jar:file:///'',matlabroot,''/help/toolbox/simulink/help.jar!/slref/' lower(get_param(gcbh,'Blocktype')) '.html''], ''-helpbrowser''),end'])
      mask Display: plot([0.2 0.35 NaN 0.65 0.8],[0 1 NaN 0 1]);
  PRO_AC_ProductionCycles : Subsystem  TreatAsAtomicUnit=on
  psrAlgoFlags_PRO1 : Outport  mask(TL_BusOutport){data={'#autoscaling',5,'#message',5,'#output',5,'#logdata',5,'structvar',{'type','IMPLICIT_STRUCT'},'signals',{{'',{'b8TriggerFlag_PR01';'b8InterruptFlag_PRO1';'b8PreActivationFlag_PRO1';'b8PreConditionsFlag_PRO1';'u8TriggeringSource_PRO1'}}},'date',736811.3265981829}}
      settings: DeleteFcn=if exist('delete_tlblock','file')==2,delete_tlblock(gcbh);end  OpenFcn=if exist('tl_open_blockdlg','file')==2,tl_open_blockdlg(gcbh);else,open_system(gcbh,'parameter');end
      settings: CopyFcn=|
      | if exist('tl_reset_reviewflag','file')==2
      |     tl_reset_reviewflag(gcbh);
      | end
      | if exist('tl_check_ports','file')
      |     tl_check_ports(gcbh);
      | end
      settings: NameChangeFcn=|
      | if exist('rename_tlblock','file')==2,rename_tlblock(gcbh);end
      | if exist('tl_check_ports','file'), tl_check_ports(gcbh); end
      mask Help: eval(['if exist(''tl_online_help'',''file'') == 2, tl_online_help(''Topic'',''TL_Outport''),else, web([''jar:file:///'',matlabroot,''/help/toolbox/simulink/help.jar!/slref/' lower(get_param(gcbh,'Blocktype')) '.html''], ''-helpbrowser''),end'])
      mask Display: plot([0.2 0.35 NaN 0.65 0.8],[0 1 NaN 0 1]);
  psrAlgoFlags_PRO2 : Outport  Port=2  mask(TL_BusOutport){data={'#autoscaling',5,'#message',5,'#output',5,'#logdata',5,'structvar',{'type','IMPLICIT_STRUCT'},'signals',{{'',{'b8TriggerFlag_PRO2';'b8InterruptFlag_PRO2';'b8ActivationFlag_PRO2';'b8PreConditionsFlag_PRO2';'u8TriggeringSource_PRO2'}}},'date',736811.32659978012}}
      settings: DeleteFcn=if exist('delete_tlblock','file')==2,delete_tlblock(gcbh);end  OpenFcn=if exist('tl_open_blockdlg','file')==2,tl_open_blockdlg(gcbh);else,open_system(gcbh,'parameter');end
      settings: CopyFcn=|
      | if exist('tl_reset_reviewflag','file')==2
      |     tl_reset_reviewflag(gcbh);
      | end
      | if exist('tl_check_ports','file')
      |     tl_check_ports(gcbh);
      | end
      settings: NameChangeFcn=|
      | if exist('rename_tlblock','file')==2,rename_tlblock(gcbh);end
      | if exist('tl_check_ports','file'), tl_check_ports(gcbh); end
      mask Help: eval(['if exist(''tl_online_help'',''file'') == 2, tl_online_help(''Topic'',''TL_Outport''),else, web([''jar:file:///'',matlabroot,''/help/toolbox/simulink/help.jar!/slref/' lower(get_param(gcbh,'Blocktype')) '.html''], ''-helpbrowser''),end'])
      mask Display: plot([0.2 0.35 NaN 0.65 0.8],[0 1 NaN 0 1]);
  wires:
  u8ExecutedCycle/1 -> PRO_AC_ProductionCycles/2(u8ExecutedCycle)
  PRO_AC_ProductionCycles/1(psrAlgoFlags_PRO1) -> psrAlgoFlags_PRO1/1
  b8DTCInhibition/1 -> PRO_AC_ProductionCycles/3(b8InhibitionOfBeltFunctionsByInternalFailure)
  b8DTCAbortion/1 -> PRO_AC_ProductionCycles/4(b8AbortionOfBeltFunctionsByInternalFailure)
  prrDiagRequestCycle/1 -> PRO_AC_ProductionCycles/1(prrDiagRequestCycle)
  PRO_AC_ProductionCycles/2(psrAlgoFlags_PRO2) -> psrAlgoFlags_PRO2/1
  u8FailureStatus/1 -> PRO_AC_ProductionCycles/5(u8FailureStatus)

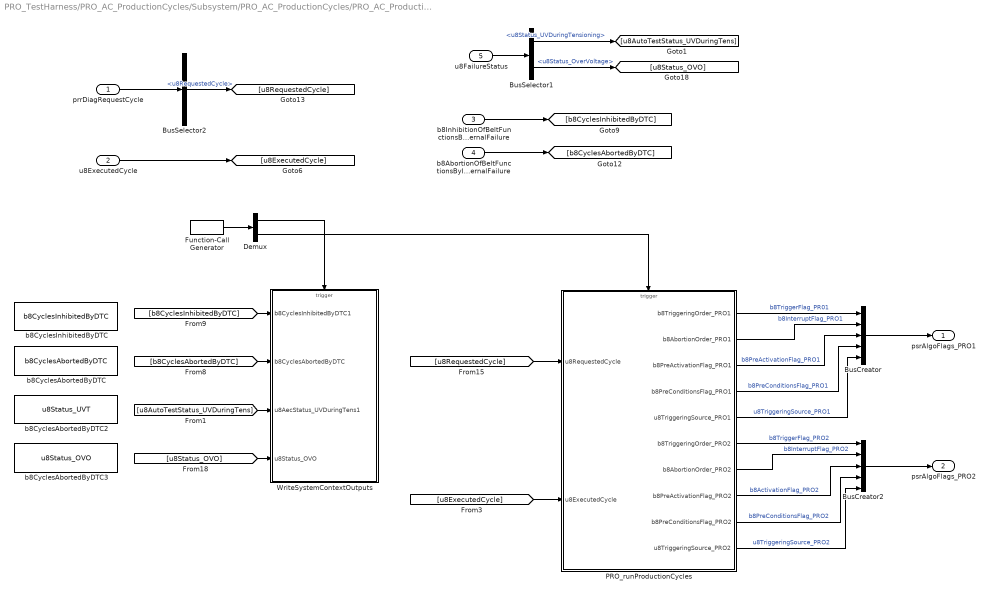
== system PRO_TestHarness/PRO_AC_ProductionCycles/Subsystem/PRO_AC_ProductionCycles/PRO_AC_ProductionCycles ==
  prrDiagRequestCycle : Inport  OutDataTypeStr=uint8
  u8ExecutedCycle : Inport  Port=2  OutDataTypeStr=uint8
  b8InhibitionOfBeltFunctionsByInternalFailure : Inport  Port=3
  b8AbortionOfBeltFunctionsByInternalFailure : Inport  Port=4
  u8FailureStatus : Inport  Port=5  OutDataTypeStr=uint8
  BusCreator : BusCreator  Inputs=5
  BusCreator2 : BusCreator  Inputs=5
  BusSelector1 : BusSelector  OutputSignals=u8Status_UVDuringTensioning,u8Status_OverVoltage
  BusSelector2 : BusSelector  OutputSignals=u8RequestedCycle
  Demux : Demux  RequirementInfo={} %GIDa_cc0bf185_c68b_4167_a31f_0b385e0fda83  Outputs=2
  Function-Call Generator : simulink/Ports & Subsystems/Function-Call Generator  RequirementInfo={} %GIDa_e54d3b28_b1f7_4169_9279_b2b1d18f1dd6  sample_time=-1  numberOfIterations=1
  PRO_runProductionCycles : Subsystem  TreatAsAtomicUnit=on
  WriteSystemContextOutputs : Subsystem
  b8CyclesAbortedByDTC : DataStoreMemory  DataStoreName=b8CyclesAbortedByDTC  ReadBeforeWriteMsg=warning  WriteAfterWriteMsg=warning  WriteAfterReadMsg=warning  InitialValue=ddv('BFD/b8CyclesAbortedByDTC')  mask(TL_DataStoreMemory){data={'output',{'variable','BFD/b8CyclesAbortedByDTC'},'date',735893.5781467593}}
      settings: CopyFcn=if exist('tl_reset_reviewflag') == 2, tl_reset_reviewflag(gcbh); end  DeleteFcn=if exist('delete_tlblock','file')==2,delete_tlblock(gcbh);end  NameChangeFcn=if exist('rename_tlblock','file')==2,rename_tlblock(gcbh);end  OpenFcn=if exist('tl_open_blockdlg','file')==2,tl_open_blockdlg(gcbh);else,open_system(gcbh,'parameter');end
      mask Help: eval(['if exist(''tl_online_help'',''file'') == 2, tl_online_help(''Topic'',''TL_DataStoreMemory''),else, web([''jar:file:///'',matlabroot,''/help/toolbox/simulink/help.jar!/slref/' lower(get_param(gcbh,'Blocktype')) '.html''], ''-helpbrowser''),end'])
      mask Display: plot([-0.05, 1.05, NaN, -0.05, 1.05],[.01, .01, NaN, .99, .99])
  b8CyclesAbortedByDTC2 : DataStoreMemory  DataStoreName=u8Status_UVT  ReadBeforeWriteMsg=warning  WriteAfterWriteMsg=warning  WriteAfterReadMsg=warning  InitialValue=ddv('BFD/u8Status_UVT')  mask(TL_DataStoreMemory){data={'output',{'variable','BFD/u8Status_UVT'},'date',736231.39883344912}}
      settings: CopyFcn=if exist('tl_reset_reviewflag') == 2, tl_reset_reviewflag(gcbh); end  DeleteFcn=if exist('delete_tlblock','file')==2,delete_tlblock(gcbh);end  NameChangeFcn=if exist('rename_tlblock','file')==2,rename_tlblock(gcbh);end  OpenFcn=if exist('tl_open_blockdlg','file')==2,tl_open_blockdlg(gcbh);else,open_system(gcbh,'parameter');end
      mask Help: eval(['if exist(''tl_online_help'',''file'') == 2, tl_online_help(''Topic'',''TL_DataStoreMemory''),else, web([''jar:file:///'',matlabroot,''/help/toolbox/simulink/help.jar!/slref/' lower(get_param(gcbh,'Blocktype')) '.html''], ''-helpbrowser''),end'])
      mask Display: plot([-0.05, 1.05, NaN, -0.05, 1.05],[.01, .01, NaN, .99, .99])
  b8CyclesAbortedByDTC3 : DataStoreMemory  DataStoreName=u8Status_OVO  ReadBeforeWriteMsg=warning  WriteAfterWriteMsg=warning  WriteAfterReadMsg=warning  InitialValue=ddv('BFD/u8Status_OVO')  mask(TL_DataStoreMemory){data={'output',{'variable','BFD/u8Status_OVO'},'date',735987.71405915509}}
      settings: CopyFcn=if exist('tl_reset_reviewflag') == 2, tl_reset_reviewflag(gcbh); end  DeleteFcn=if exist('delete_tlblock','file')==2,delete_tlblock(gcbh);end  NameChangeFcn=if exist('rename_tlblock','file')==2,rename_tlblock(gcbh);end  OpenFcn=if exist('tl_open_blockdlg','file')==2,tl_open_blockdlg(gcbh);else,open_system(gcbh,'parameter');end
      mask Help: eval(['if exist(''tl_online_help'',''file'') == 2, tl_online_help(''Topic'',''TL_DataStoreMemory''),else, web([''jar:file:///'',matlabroot,''/help/toolbox/simulink/help.jar!/slref/' lower(get_param(gcbh,'Blocktype')) '.html''], ''-helpbrowser''),end'])
      mask Display: plot([-0.05, 1.05, NaN, -0.05, 1.05],[.01, .01, NaN, .99, .99])
  b8CyclesInhibitedByDTC : DataStoreMemory  DataStoreName=b8CyclesInhibitedByDTC  ReadBeforeWriteMsg=warning  WriteAfterWriteMsg=warning  WriteAfterReadMsg=warning  InitialValue=ddv('BFD/b8CyclesInhibitedByDTC')  mask(TL_DataStoreMemory){data={'output',{'variable','BFD/b8CyclesInhibitedByDTC'},'date',735893.57807276619}}
      settings: CopyFcn=if exist('tl_reset_reviewflag') == 2, tl_reset_reviewflag(gcbh); end  DeleteFcn=if exist('delete_tlblock','file')==2,delete_tlblock(gcbh);end  NameChangeFcn=if exist('rename_tlblock','file')==2,rename_tlblock(gcbh);end  OpenFcn=if exist('tl_open_blockdlg','file')==2,tl_open_blockdlg(gcbh);else,open_system(gcbh,'parameter');end
      mask Help: eval(['if exist(''tl_online_help'',''file'') == 2, tl_online_help(''Topic'',''TL_DataStoreMemory''),else, web([''jar:file:///'',matlabroot,''/help/toolbox/simulink/help.jar!/slref/' lower(get_param(gcbh,'Blocktype')) '.html''], ''-helpbrowser''),end'])
      mask Display: plot([-0.05, 1.05, NaN, -0.05, 1.05],[.01, .01, NaN, .99, .99])
  psrAlgoFlags_PRO1 : Outport
  psrAlgoFlags_PRO2 : Outport  Port=2
  wires:
  [u8ExecutedCycle] -> PRO_runProductionCycles/2(u8ExecutedCycle)
  PRO_runProductionCycles/2(b8AbortionOrder_PRO1) -> BusCreator/2  "b8InterruptFlag_PRO1"
  u8ExecutedCycle/1 -> [u8ExecutedCycle]
  PRO_runProductionCycles/1(b8TriggeringOrder_PRO1) -> BusCreator/1  "b8TriggerFlag_PR01"
  b8InhibitionOfBeltFunctionsByInternalFailure/1 -> [b8CyclesInhibitedByDTC]
  b8AbortionOfBeltFunctionsByInternalFailure/1 -> [b8CyclesAbortedByDTC]
  Function-Call Generator/1 -> Demux/1
  Demux/1 -> WriteSystemContextOutputs/Trigger
  Demux/2 -> PRO_runProductionCycles/Trigger
  PRO_runProductionCycles/3(b8PreActivationFlag_PRO1) -> BusCreator/3  "b8PreActivationFlag_PRO1"
  PRO_runProductionCycles/4(b8PreConditionsFlag_PRO1) -> BusCreator/4  "b8PreConditionsFlag_PRO1"
  PRO_runProductionCycles/5(u8TriggeringSource_PRO1) -> BusCreator/5  "u8TriggeringSource_PRO1"
  [u8RequestedCycle] -> PRO_runProductionCycles/1(u8RequestedCycle)
  [b8CyclesInhibitedByDTC] -> WriteSystemContextOutputs/1(b8CyclesInhibitedByDTC1)
  [b8CyclesAbortedByDTC] -> WriteSystemContextOutputs/2(b8CyclesAbortedByDTC)
  BusSelector2/1 -> [u8RequestedCycle]  "<u8RequestedCycle>"
  prrDiagRequestCycle/1 -> BusSelector2/1
  BusCreator2/1 -> psrAlgoFlags_PRO2/1
  PRO_runProductionCycles/6(b8TriggeringOrder_PRO2) -> BusCreator2/1  "b8TriggerFlag_PRO2"
  PRO_runProductionCycles/7(b8AbortionOrder_PRO2) -> BusCreator2/2  "b8InterruptFlag_PRO2"
  PRO_runProductionCycles/8(b8PreActivationFlag_PRO2) -> BusCreator2/3  "b8ActivationFlag_PRO2"
  PRO_runProductionCycles/9(b8PreConditionsFlag_PRO2) -> BusCreator2/4  "b8PreConditionsFlag_PRO2"
  PRO_runProductionCycles/10(u8TriggeringSource_PRO2) -> BusCreator2/5  "u8TriggeringSource_PRO2"
  BusCreator/1 -> psrAlgoFlags_PRO1/1
  [u8AutoTestStatus_UVDuringTens] -> WriteSystemContextOutputs/3(u8AecStatus_UVDuringTens1)
  [u8Status_OVO] -> WriteSystemContextOutputs/4(u8Status_OVO)
  BusSelector1/1 -> [u8AutoTestStatus_UVDuringTens]  "<u8Status_UVDuringTensioning>"
  BusSelector1/2 -> [u8Status_OVO]  "<u8Status_OverVoltage>"
  u8FailureStatus/1 -> BusSelector1/1
